simulink model "CMOS_Kernel_Memory_Sync"  (R2023b)
settings: Solver=VariableStepAuto  StartTime=0.0  StopTime=30000000  RelTol=1e-3
values from neighbouring files (symbols this model uses):
  AmountOfPixelsPerScanline = 400    [Kernel_Setup_Script.m]
  AmountOfRamBlocksScanlines = 5    [Kernel_Setup_Script.m]
  AmountOfRamBlocksScanlinesOffset = AmountOfRamBlocksScanlines - 1    (= 4)    [Kernel_Setup_Script.m]
  AmountOfScanlinePixels = 73700    [Kernel_Setup_Script.m]
  AmountOfScanlinePixelsOffset = AmountOfScanlinePixels - 1    (= 73699)    [Kernel_Setup_Script.m]
  AmountOfScanlines = 1100    [Kernel_Setup_Script.m]
  AmountOfScanlinesOffset = AmountOfScanlines - 1    (= 1099)    [Kernel_Setup_Script.m]
  AOPPK_Off = AmountOfPixelsPerScanline - 1    (= 399)    [Kernel_Setup_Script.m]
  AOPPS_Off = AmountOfPixelsPerScanline - 1    (= 399)    [Kernel_Setup_Script.m]
  FramePackOff_0 = FramePackOff_0 - ScanlineFifoCheck    [Kernel_Setup_Script.m]
  FramePackOff_1 = FramePackOff_1 - ScanlineFifoCheck    [Kernel_Setup_Script.m]
  FramePackOff_2 = FramePackOff_2 - ScanlineFifoCheck    [Kernel_Setup_Script.m]
  FramePackOff_3 = FramePackOff_3 - ScanlineFifoCheck    [Kernel_Setup_Script.m]
  FramePackOff_4 = FramePackOff_4 - ScanlineFifoCheck    [Kernel_Setup_Script.m]
  FramePackOff_5 = FramePackOff_5 - ScanlineFifoCheck    [Kernel_Setup_Script.m]
  KernelPackOff_0 = KernelPackOff_0 - KernelBitsPerRow    [Kernel_Setup_Script.m]
  KernelPackOff_1 = KernelPackOff_1 - KernelBitsPerRow    [Kernel_Setup_Script.m]
  KernelPackOff_2 = KernelPackOff_2 - KernelBitsPerRow    [Kernel_Setup_Script.m]
  KernelPackOff_3 = KernelPackOff_3 - KernelBitsPerRow    [Kernel_Setup_Script.m]
  Slice59DownTo48Top = (MsbOffset - (ScanlinePixelBitSizeController*1))    (= 59)    [Kernel_Setup_Script.m]
  Slice71DownTo60Top = (MsbOffset - (ScanlinePixelBitSizeController*0))    (= 71)    [Kernel_Setup_Script.m]
  TotalSectionsForFrames = AmountOfScanlines/AmountOfRamBlocksScanlines    (= 220)    [Kernel_Setup_Script.m]
  UltraRamRows = AmountOfPixelsPerScanline/ScanlineFifoCheck    [Kernel_Setup_Script.m]
  UltraRamRowsCeil = ceil(AmountOfPixelsPerScanline/ScanlineFifoCheck)    [Kernel_Setup_Script.m]
  UltraRamRowsKernel = AmountOfPixelsPerScanline/KernelBitsPerRow    (= 100)    [Kernel_Setup_Script.m]
  UltraRamRowsKernelCeil = ceil(AmountOfPixelsPerScanline/KernelBitsPerRow)    [Kernel_Setup_Script.m]
  UltraRamRowsMemorySectionOffset = UltraRamRowsCeil*AmountOfRamBlocksScanlines    [Kernel_Setup_Script.m]
  UltraRamRowsOffset = UltraRamRowsCeil - 1    [Kernel_Setup_Script.m]
undefined symbols (not defined in the file or in its folder): c, Down, sfvc784, Up, xck26
libraries: hdlBasic x4512, vmcUtilities x1
(part 6 of 39)

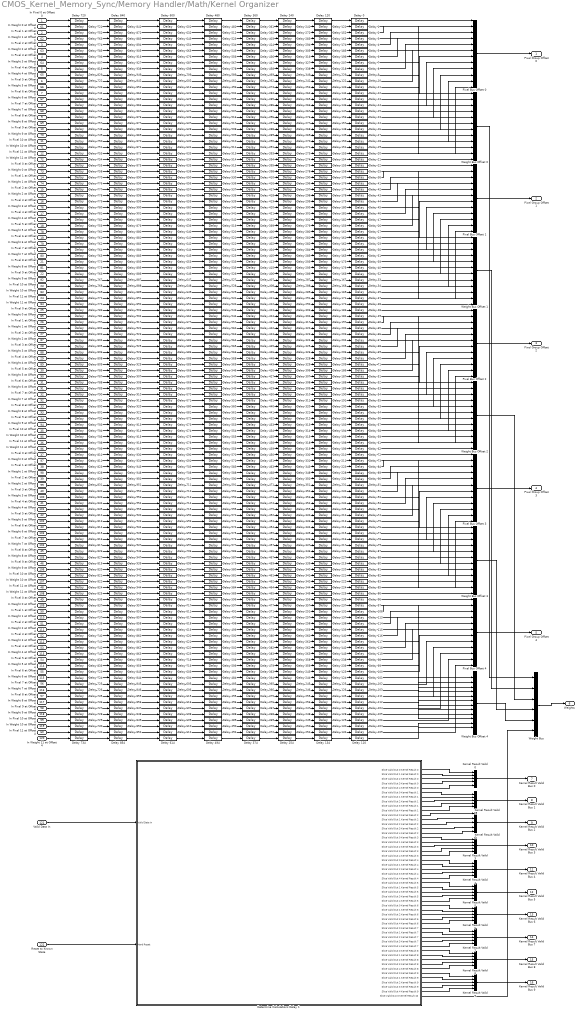
== system CMOS_Kernel_Memory_Sync/Memory Handler/Math/Kernel Organizer ==
  In Pixel 0 at Offset 0 : Inport
  In Pixel 1 at Offset 0 : Inport  Port=2
  In Pixel 2 at Offset 0 : Inport  Port=3
  In Pixel 3 at Offset 0 : Inport  Port=4
  In Pixel 4 at Offset 0 : Inport  Port=5
  In Pixel 5 at Offset 0 : Inport  Port=6
  In Pixel 6 at Offset 0 : Inport  Port=7
  In Pixel 7 at Offset 0 : Inport  Port=8
  In Pixel 8 at Offset 0 : Inport  Port=9
  In Pixel 9 at Offset 0 : Inport  Port=10
  In Pixel 10 at Offset 0 : Inport  Port=11
  In Pixel 11 at Offset 0 : Inport  Port=12
  In Pixel 0 at Offset 1 : Inport  Port=13
  In Pixel 1 at Offset 1 : Inport  Port=14
  In Pixel 2 at Offset 1 : Inport  Port=15
  In Pixel 3 at Offset 1 : Inport  Port=16
  In Pixel 4 at Offset 1 : Inport  Port=17
  In Pixel 5 at Offset 1 : Inport  Port=18
  In Pixel 6 at Offset 1 : Inport  Port=19
  In Pixel 7 at Offset 1 : Inport  Port=20
  In Pixel 8 at Offset 1 : Inport  Port=21
  In Pixel 9 at Offset 1 : Inport  Port=22
  In Pixel 10 at Offset 1 : Inport  Port=23
  In Pixel 11 at Offset 1 : Inport  Port=24
  In Pixel 0 at Offset 2 : Inport  Port=25
  In Pixel 1 at Offset 2 : Inport  Port=26
  In Pixel 2 at Offset 2 : Inport  Port=27
  In Pixel 3 at Offset 2 : Inport  Port=28
  In Pixel 4 at Offset 2 : Inport  Port=29
  In Pixel 5 at Offset 2 : Inport  Port=30
  In Pixel 6 at Offset 2 : Inport  Port=31
  In Pixel 7 at Offset 2 : Inport  Port=32
  In Pixel 8 at Offset 2 : Inport  Port=33
  In Pixel 9 at Offset 2 : Inport  Port=34
  In Pixel 10 at Offset 2 : Inport  Port=35
  In Pixel 11 at Offset 2 : Inport  Port=36
  In Pixel 0 at Offset 3 : Inport  Port=37
  In Pixel 1 at Offset 3 : Inport  Port=38
  In Pixel 2 at Offset 3 : Inport  Port=39
  In Pixel 3 at Offset 3 : Inport  Port=40
  In Pixel 4 at Offset 3 : Inport  Port=41
  In Pixel 5 at Offset 3 : Inport  Port=42
  In Pixel 6 at Offset 3 : Inport  Port=43
  In Pixel 7 at Offset 3 : Inport  Port=44
  In Pixel 8 at Offset 3 : Inport  Port=45
  In Pixel 9 at Offset 3 : Inport  Port=46
  In Pixel 10 at Offset 3 : Inport  Port=47
  In Pixel 11 at Offset 3 : Inport  Port=48
  In Pixel 0 at Offset 4 : Inport  Port=49
  In Pixel 1 at Offset 4 : Inport  Port=50
  In Pixel 2 at Offset 4 : Inport  Port=51
  In Pixel 3 at Offset 4 : Inport  Port=52
  In Pixel 4 at Offset 4 : Inport  Port=53
  In Pixel 5 at Offset 4 : Inport  Port=54
  In Pixel 6 at Offset 4 : Inport  Port=55
  In Pixel 7 at Offset 4 : Inport  Port=56
  In Pixel 8 at Offset 4 : Inport  Port=57
  In Pixel 9 at Offset 4 : Inport  Port=58
  In Pixel 10 at Offset 4 : Inport  Port=59
  In Pixel 11 at Offset 4 : Inport  Port=60
  In Weight 0 at Offset 0 : Inport  Port=61
  In Weight 1 at Offset 0 : Inport  Port=62
  In Weight 2 at Offset 0 : Inport  Port=63
  In Weight 3 at Offset 0 : Inport  Port=64
  In Weight 4 at Offset 0 : Inport  Port=65
  In Weight 5 at Offset 0 : Inport  Port=66
  In Weight 6 at Offset 0 : Inport  Port=67
  In Weight 7 at Offset 0 : Inport  Port=68
  In Weight 8 at Offset 0 : Inport  Port=69
  In Weight 9 at Offset 0 : Inport  Port=70
  In Weight 10 at Offset 0 : Inport  Port=71
  In Weight 11 at Offset 0 : Inport  Port=72
  In Weight 0 at Offset 1 : Inport  Port=73
  In Weight 1 at Offset 1 : Inport  Port=74
  In Weight 2 at Offset 1 : Inport  Port=75
  In Weight 3 at Offset 1 : Inport  Port=76
  In Weight 4 at Offset 1 : Inport  Port=77
  In Weight 5 at Offset 1 : Inport  Port=78
  In Weight 6 at Offset 1 : Inport  Port=79
  In Weight 7 at Offset 1 : Inport  Port=80
  In Weight 8 at Offset 1 : Inport  Port=81
  In Weight 9 at Offset 1 : Inport  Port=82
  In Weight 10 at Offset 1 : Inport  Port=83
  In Weight 11 at Offset 1 : Inport  Port=84
  In Weight 0 at Offset 2 : Inport  Port=85
  In Weight 1 at Offset 2 : Inport  Port=86
  In Weight 2 at Offset 2 : Inport  Port=87
  In Weight 3 at Offset 2 : Inport  Port=88
  In Weight 4 at Offset 2 : Inport  Port=89
  In Weight 5 at Offset 2 : Inport  Port=90
  In Weight 6 at Offset 2 : Inport  Port=91
  In Weight 7 at Offset 2 : Inport  Port=92
  In Weight 8 at Offset 2 : Inport  Port=93
  In Weight 9 at Offset 2 : Inport  Port=94
  In Weight 10 at Offset 2 : Inport  Port=95
  In Weight 11 at Offset 2 : Inport  Port=96
  In Weight 0 at Offset 3 : Inport  Port=97
  In Weight 1 at Offset 3 : Inport  Port=98
  In Weight 2 at Offset 3 : Inport  Port=99
  In Weight 3 at Offset 3 : Inport  Port=100
  In Weight 4 at Offset 3 : Inport  Port=101
  In Weight 5 at Offset 3 : Inport  Port=102
  In Weight 6 at Offset 3 : Inport  Port=103
  In Weight 7 at Offset 3 : Inport  Port=104
  In Weight 8 at Offset 3 : Inport  Port=105
  In Weight 9 at Offset 3 : Inport  Port=106
  In Weight 10 at Offset 3 : Inport  Port=107
  In Weight 11 at Offset 3 : Inport  Port=108
  In Weight 0 at Offset 4 : Inport  Port=109
  In Weight 1 at Offset 4 : Inport  Port=110
  In Weight 2 at Offset 4 : Inport  Port=111
  In Weight 3 at Offset 4 : Inport  Port=112
  In Weight 4 at Offset 4 : Inport  Port=113
  In Weight 5 at Offset 4 : Inport  Port=114
  In Weight 6 at Offset 4 : Inport  Port=115
  In Weight 7 at Offset 4 : Inport  Port=116
  In Weight 8 at Offset 4 : Inport  Port=117
  In Weight 9 at Offset 4 : Inport  Port=118
  In Weight 10 at Offset 4 : Inport  Port=119
  In Weight 11 at Offset 4 : Inport  Port=120
  Valid Data In : Inport  Port=121
  Reset to Known State : Inport  Port=122
  Delay {0..959} (960 alike) : hdlBasic/Delay  rst=off  en=off  latency=1  reg_retiming=off  XmcBlockStatus=1  maskContainerNames=group1  block_type=delay  block_config=sysgen:Delay_config
  Determine Calculations Delay 1 : Subsystem
  Kernel Result Valid {0..9} (10 alike) : BusCreator  Inputs=5
  Pixel Bus Offset {0..4} (5 alike) : BusCreator  Inputs=12
  Weight Bus : BusCreator  Inputs=6
  Weight Bus Offset {0..4} (5 alike) : BusCreator  Inputs=12
  Pixel Group Offset 0 : Outport
  Pixel Group Offset 1 : Outport  Port=2
  Pixel Group Offset 2 : Outport  Port=3
  Pixel Group Offset 3 : Outport  Port=4
  Pixel Group Offset 4 : Outport  Port=5
  Weights : Outport  Port=6
  Kernel Result Valid Bus 0 : Outport  Port=7
  Kernel Result Valid Bus 1 : Outport  Port=8
  Kernel Result Valid Bus 2 : Outport  Port=9
  Kernel Result Valid Bus 3 : Outport  Port=10
  Kernel Result Valid Bus 4 : Outport  Port=11
  Kernel Result Valid Bus 5 : Outport  Port=12
  Kernel Result Valid Bus 6 : Outport  Port=13
  Kernel Result Valid Bus 7 : Outport  Port=14
  Kernel Result Valid Bus 8 : Outport  Port=15
  Kernel Result Valid Bus 9 : Outport  Port=16
  wires:
  Delay 3/1 -> Weight Bus Offset 0/2
  Delay 2/1 -> Pixel Bus Offset 0/2
  Delay 5/1 -> Weight Bus Offset 0/3
  Delay 7/1 -> Weight Bus Offset 0/4
  Delay 6/1 -> Pixel Bus Offset 0/4
  Delay 4/1 -> Pixel Bus Offset 0/3
  Delay 9/1 -> Weight Bus Offset 0/5
  Delay 11/1 -> Weight Bus Offset 0/6
  Delay 10/1 -> Pixel Bus Offset 0/6
  Delay 8/1 -> Pixel Bus Offset 0/5
  Delay 12/1 -> Pixel Bus Offset 0/7
  Delay 13/1 -> Weight Bus Offset 0/7
  Delay 15/1 -> Weight Bus Offset 0/8
  Delay 14/1 -> Pixel Bus Offset 0/8
  Delay 23/1 -> Pixel Bus Offset 0/9
  Delay 16/1 -> Pixel Bus Offset 0/10
  Delay 17/1 -> Weight Bus Offset 0/10
  Delay 19/1 -> Weight Bus Offset 0/11
  Delay 20/1 -> Pixel Bus Offset 0/12
  Delay 21/1 -> Weight Bus Offset 0/12
  Delay 24/1 -> Weight Bus Offset 0/9
  Delay 18/1 -> Pixel Bus Offset 0/11
  Valid Data In/1 -> Determine Calculations Delay 1/1(Valid Data In)
  Determine Calculations Delay 1/1(Slice Valid Out 0 Kernel Result 0) -> Kernel Result Valid 0/1
  Determine Calculations Delay 1/2(Slice Valid Out 1 Kernel Result 0) -> Kernel Result Valid 0/2
  Determine Calculations Delay 1/3(Slice Valid Out 2 Kernel Result 0) -> Kernel Result Valid 0/3
  Determine Calculations Delay 1/4(Slice Valid Out 3 Kernel Result 0) -> Kernel Result Valid 0/4
  Determine Calculations Delay 1/5(Slice Valid Out 4 Kernel Result 0) -> Kernel Result Valid 0/5
  Determine Calculations Delay 1/10(Slice Valid Out 4 Kernel Result 1) -> Kernel Result Valid 1/5
  Determine Calculations Delay 1/6(Slice Valid Out 0 Kernel Result 1) -> Kernel Result Valid 1/1
  Determine Calculations Delay 1/7(Slice Valid Out 1 Kernel Result 1) -> Kernel Result Valid 1/2
  Determine Calculations Delay 1/9(Slice Valid Out 3 Kernel Result 1) -> Kernel Result Valid 1/4
  Determine Calculations Delay 1/8(Slice Valid Out 2 Kernel Result 1) -> Kernel Result Valid 1/3
  Determine Calculations Delay 1/15(Slice Valid Out 4 Kernel Result 2) -> Kernel Result Valid 2/5
  Determine Calculations Delay 1/19(Slice Valid Out 3 Kernel Result 3) -> Kernel Result Valid 3/4
  Determine Calculations Delay 1/17(Slice Valid Out 1 Kernel Result 3) -> Kernel Result Valid 3/2
  Determine Calculations Delay 1/16(Slice Valid Out 0 Kernel Result 3) -> Kernel Result Valid 3/1
  Determine Calculations Delay 1/11(Slice Valid Out 0 Kernel Result 2) -> Kernel Result Valid 2/1
  Determine Calculations Delay 1/12(Slice Valid Out 1 Kernel Result 2) -> Kernel Result Valid 2/2
  Determine Calculations Delay 1/18(Slice Valid Out 2 Kernel Result 3) -> Kernel Result Valid 3/3
  Determine Calculations Delay 1/14(Slice Valid Out 3 Kernel Result 2) -> Kernel Result Valid 2/4
  Determine Calculations Delay 1/20(Slice Valid Out 4 Kernel Result 3) -> Kernel Result Valid 3/5
  Determine Calculations Delay 1/13(Slice Valid Out 2 Kernel Result 2) -> Kernel Result Valid 2/3
  Determine Calculations Delay 1/25(Slice Valid Out 4 Kernel Result 4) -> Kernel Result Valid 4/5
  Determine Calculations Delay 1/21(Slice Valid Out 0 Kernel Result 4) -> Kernel Result Valid 4/1
  Determine Calculations Delay 1/22(Slice Valid Out 1 Kernel Result 4) -> Kernel Result Valid 4/2
  Determine Calculations Delay 1/24(Slice Valid Out 3 Kernel Result 4) -> Kernel Result Valid 4/4
  Determine Calculations Delay 1/23(Slice Valid Out 2 Kernel Result 4) -> Kernel Result Valid 4/3
  Delay 0/1 -> Pixel Bus Offset 0/1
  Delay 1/1 -> Weight Bus Offset 0/1
  Delay 43/1 -> Weight Bus Offset 1/3
  Delay 37/1 -> Pixel Bus Offset 1/12
  Delay 35/1 -> Weight Bus Offset 1/11
  Delay 46/1 -> Pixel Bus Offset 1/5
  Delay 33/1 -> Weight Bus Offset 1/10
  Delay 40/1 -> Weight Bus Offset 1/9
  Delay 28/1 -> Pixel Bus Offset 1/7
  Delay 47/1 -> Weight Bus Offset 1/5
  Delay 22/1 -> Pixel Bus Offset 1/1
  Delay 25/1 -> Weight Bus Offset 1/1
  Delay 38/1 -> Weight Bus Offset 1/12
  Delay 30/1 -> Pixel Bus Offset 1/8
  Delay 36/1 -> Pixel Bus Offset 1/2
  Delay 45/1 -> Weight Bus Offset 1/4
  Delay 42/1 -> Pixel Bus Offset 1/3
  Delay 27/1 -> Weight Bus Offset 1/6
  Delay 39/1 -> Pixel Bus Offset 1/9
  Delay 29/1 -> Weight Bus Offset 1/7
  Delay 34/1 -> Pixel Bus Offset 1/11
  Delay 26/1 -> Pixel Bus Offset 1/6
  Delay 31/1 -> Weight Bus Offset 1/8
  Delay 44/1 -> Pixel Bus Offset 1/4
  Delay 41/1 -> Weight Bus Offset 1/2
  Delay 32/1 -> Pixel Bus Offset 1/10
  Delay 67/1 -> Weight Bus Offset 2/3
  Delay 61/1 -> Pixel Bus Offset 2/12
  Delay 59/1 -> Weight Bus Offset 2/11
  Delay 70/1 -> Pixel Bus Offset 2/5
  Delay 57/1 -> Weight Bus Offset 2/10
  Delay 64/1 -> Weight Bus Offset 2/9
  Delay 52/1 -> Pixel Bus Offset 2/7
  Delay 71/1 -> Weight Bus Offset 2/5
  Delay 48/1 -> Pixel Bus Offset 2/1
  Delay 49/1 -> Weight Bus Offset 2/1
  Delay 62/1 -> Weight Bus Offset 2/12
  Delay 54/1 -> Pixel Bus Offset 2/8
  Delay 60/1 -> Pixel Bus Offset 2/2
  Delay 69/1 -> Weight Bus Offset 2/4
  Delay 66/1 -> Pixel Bus Offset 2/3
  Delay 51/1 -> Weight Bus Offset 2/6
  Delay 63/1 -> Pixel Bus Offset 2/9
  Delay 53/1 -> Weight Bus Offset 2/7
  Delay 58/1 -> Pixel Bus Offset 2/11
  Delay 50/1 -> Pixel Bus Offset 2/6
  Delay 55/1 -> Weight Bus Offset 2/8
  Delay 68/1 -> Pixel Bus Offset 2/4
  Delay 65/1 -> Weight Bus Offset 2/2
  Delay 56/1 -> Pixel Bus Offset 2/10
  Delay 91/1 -> Weight Bus Offset 3/3
  Delay 85/1 -> Pixel Bus Offset 3/12
  Delay 83/1 -> Weight Bus Offset 3/11
  Delay 94/1 -> Pixel Bus Offset 3/5
  Delay 81/1 -> Weight Bus Offset 3/10
  Delay 88/1 -> Weight Bus Offset 3/9
  Delay 76/1 -> Pixel Bus Offset 3/7
  Delay 95/1 -> Weight Bus Offset 3/5
  Delay 72/1 -> Pixel Bus Offset 3/1
  Delay 73/1 -> Weight Bus Offset 3/1
  Delay 86/1 -> Weight Bus Offset 3/12
  Delay 78/1 -> Pixel Bus Offset 3/8
  Delay 84/1 -> Pixel Bus Offset 3/2
  Delay 93/1 -> Weight Bus Offset 3/4
  Delay 90/1 -> Pixel Bus Offset 3/3
  Delay 75/1 -> Weight Bus Offset 3/6
  Delay 87/1 -> Pixel Bus Offset 3/9
  Delay 77/1 -> Weight Bus Offset 3/7
  Delay 82/1 -> Pixel Bus Offset 3/11
  Delay 74/1 -> Pixel Bus Offset 3/6
  Delay 79/1 -> Weight Bus Offset 3/8
  Delay 92/1 -> Pixel Bus Offset 3/4
  Delay 89/1 -> Weight Bus Offset 3/2
  Delay 80/1 -> Pixel Bus Offset 3/10
  Delay 115/1 -> Weight Bus Offset 4/3
  Delay 109/1 -> Pixel Bus Offset 4/12
  Delay 107/1 -> Weight Bus Offset 4/11
  Delay 118/1 -> Pixel Bus Offset 4/5
  Delay 105/1 -> Weight Bus Offset 4/10
  Delay 112/1 -> Weight Bus Offset 4/9
  Delay 100/1 -> Pixel Bus Offset 4/7
  Delay 119/1 -> Weight Bus Offset 4/5
  Delay 96/1 -> Pixel Bus Offset 4/1
  Delay 97/1 -> Weight Bus Offset 4/1
  Delay 110/1 -> Weight Bus Offset 4/12
  Delay 102/1 -> Pixel Bus Offset 4/8
  Delay 108/1 -> Pixel Bus Offset 4/2
  Delay 117/1 -> Weight Bus Offset 4/4
  Delay 114/1 -> Pixel Bus Offset 4/3
  Delay 99/1 -> Weight Bus Offset 4/6
  Delay 111/1 -> Pixel Bus Offset 4/9
  Delay 101/1 -> Weight Bus Offset 4/7
  Delay 106/1 -> Pixel Bus Offset 4/11
  Delay 98/1 -> Pixel Bus Offset 4/6
  Delay 103/1 -> Weight Bus Offset 4/8
  Delay 116/1 -> Pixel Bus Offset 4/4
  Delay 113/1 -> Weight Bus Offset 4/2
  Delay 104/1 -> Pixel Bus Offset 4/10
  Pixel Bus Offset 0/1 -> Pixel Group Offset 0/1
  Pixel Bus Offset 1/1 -> Pixel Group Offset 1/1
  Pixel Bus Offset 2/1 -> Pixel Group Offset 2/1
  Pixel Bus Offset 3/1 -> Pixel Group Offset 3/1
  Pixel Bus Offset 4/1 -> Pixel Group Offset 4/1
  Kernel Result Valid 0/1 -> Kernel Result Valid Bus 0/1
  Kernel Result Valid 1/1 -> Kernel Result Valid Bus 1/1
  Kernel Result Valid 3/1 -> Kernel Result Valid Bus 3/1
  Kernel Result Valid 2/1 -> Kernel Result Valid Bus 2/1
  Kernel Result Valid 4/1 -> Kernel Result Valid Bus 4/1
  Delay 171/1 -> Delay 37/1
  Delay 189/1 -> Delay 53/1
  Delay 190/1 -> Delay 54/1
  Delay 187/1 -> Delay 51/1
  Delay 188/1 -> Delay 52/1
  Delay 137/1 -> Delay 113/1
  Delay 157/1 -> Delay 24/1
  Delay 152/1 -> Delay 2/1
  Delay 150/1 -> Delay 18/1
  Delay 143/1 -> Delay 119/1
  Delay 144/1 -> Delay 12/1
  Delay 145/1 -> Delay 13/1
  Delay 146/1 -> Delay 14/1
  Delay 147/1 -> Delay 15/1
  Delay 148/1 -> Delay 16/1
  Delay 120/1 -> Delay 0/1
  Delay 121/1 -> Delay 1/1
  Delay 122/1 -> Delay 10/1
  Delay 123/1 -> Delay 100/1
  Delay 124/1 -> Delay 101/1
  Delay 126/1 -> Delay 103/1
  Delay 125/1 -> Delay 102/1
  Delay 128/1 -> Delay 105/1
  Delay 129/1 -> Delay 106/1
  Delay 131/1 -> Delay 108/1
  Delay 130/1 -> Delay 107/1
  Delay 134/1 -> Delay 110/1
  Delay 132/1 -> Delay 109/1
  Delay 133/1 -> Delay 11/1
  Delay 151/1 -> Delay 19/1
  Delay 135/1 -> Delay 111/1
  Delay 141/1 -> Delay 117/1
  Delay 136/1 -> Delay 112/1
  Delay 160/1 -> Delay 27/1
  Delay 219/1 -> Delay 80/1
  Delay 185/1 -> Delay 5/1
  Delay 191/1 -> Delay 55/1
  Delay 182/1 -> Delay 47/1
  Delay 183/1 -> Delay 48/1
  Delay 184/1 -> Delay 49/1
  Delay 179/1 -> Delay 44/1
  Delay 178/1 -> Delay 43/1
  Delay 180/1 -> Delay 45/1
  Delay 173/1 -> Delay 39/1
  Delay 174/1 -> Delay 4/1
  Delay 175/1 -> Delay 40/1
  Delay 176/1 -> Delay 41/1
  Delay 177/1 -> Delay 42/1
  Delay 208/1 -> Delay 70/1
  Delay 207/1 -> Delay 7/1
  Delay 200/1 -> Delay 63/1
  Delay 214/1 -> Delay 76/1
  Delay 215/1 -> Delay 77/1
  Delay 217/1 -> Delay 79/1
  Delay 211/1 -> Delay 73/1
  Delay 209/1 -> Delay 71/1
  Delay 210/1 -> Delay 72/1
  Delay 212/1 -> Delay 74/1
  Delay 213/1 -> Delay 75/1
  Delay 192/1 -> Delay 56/1
  Delay 158/1 -> Delay 25/1
  Delay 142/1 -> Delay 118/1
  Delay 138/1 -> Delay 114/1
  Delay 140/1 -> Delay 116/1
  Delay 201/1 -> Delay 64/1
  Delay 203/1 -> Delay 66/1
  Delay 204/1 -> Delay 67/1
  Delay 205/1 -> Delay 68/1
  Delay 206/1 -> Delay 69/1
  Delay 216/1 -> Delay 78/1
  Delay 220/1 -> Delay 81/1
  Delay 199/1 -> Delay 62/1
  Delay 202/1 -> Delay 65/1
  Delay 186/1 -> Delay 50/1
  Delay 193/1 -> Delay 57/1
  Delay 194/1 -> Delay 58/1
  Delay 195/1 -> Delay 59/1
  Delay 196/1 -> Delay 6/1
  Delay 197/1 -> Delay 60/1
  Delay 198/1 -> Delay 61/1
  Delay 226/1 -> Delay 87/1
  Delay 224/1 -> Delay 85/1
  Delay 227/1 -> Delay 88/1
  Delay 225/1 -> Delay 86/1
  Delay 229/1 -> Delay 9/1
  Delay 231/1 -> Delay 91/1
  Delay 228/1 -> Delay 89/1
  Delay 230/1 -> Delay 90/1
  Delay 233/1 -> Delay 93/1
  Delay 232/1 -> Delay 92/1
  Delay 234/1 -> Delay 94/1
  Delay 235/1 -> Delay 95/1
  Delay 238/1 -> Delay 98/1
  Delay 236/1 -> Delay 96/1
  Delay 237/1 -> Delay 97/1
  Delay 239/1 -> Delay 99/1
  Delay 223/1 -> Delay 84/1
  Delay 218/1 -> Delay 8/1
  Delay 172/1 -> Delay 38/1
  Delay 169/1 -> Delay 35/1
  Delay 168/1 -> Delay 34/1
  Delay 221/1 -> Delay 82/1
  Delay 222/1 -> Delay 83/1
  Delay 170/1 -> Delay 36/1
  Delay 161/1 -> Delay 28/1
  Delay 162/1 -> Delay 29/1
  Delay 163/1 -> Delay 3/1
  Delay 165/1 -> Delay 31/1
  Delay 166/1 -> Delay 32/1
  Delay 153/1 -> Delay 20/1
  Delay 154/1 -> Delay 21/1
  Delay 155/1 -> Delay 22/1
  Delay 156/1 -> Delay 23/1
  Delay 159/1 -> Delay 26/1
  Delay 167/1 -> Delay 33/1
  Delay 127/1 -> Delay 104/1
  Delay 149/1 -> Delay 17/1
  Delay 139/1 -> Delay 115/1
  Delay 164/1 -> Delay 30/1
  Delay 181/1 -> Delay 46/1
  Delay 279/1 -> Delay 159/1
  Delay 358/1 -> Delay 238/1
  Delay 357/1 -> Delay 237/1
  Delay 350/1 -> Delay 230/1
  Delay 351/1 -> Delay 231/1
  Delay 353/1 -> Delay 233/1
  Delay 352/1 -> Delay 232/1
  Delay 356/1 -> Delay 236/1
  Delay 320/1 -> Delay 200/1
  Delay 321/1 -> Delay 201/1
  Delay 322/1 -> Delay 202/1
  Delay 323/1 -> Delay 203/1
  Delay 324/1 -> Delay 204/1
  Delay 325/1 -> Delay 205/1
  Delay 326/1 -> Delay 206/1
  Delay 327/1 -> Delay 207/1
  Delay 328/1 -> Delay 208/1
  Delay 329/1 -> Delay 209/1
  Delay 330/1 -> Delay 210/1
  Delay 331/1 -> Delay 211/1
  Delay 333/1 -> Delay 213/1
  Delay 332/1 -> Delay 212/1
  Delay 334/1 -> Delay 214/1
  Delay 336/1 -> Delay 216/1
  Delay 335/1 -> Delay 215/1
  Delay 337/1 -> Delay 217/1
  Delay 338/1 -> Delay 218/1
  Delay 339/1 -> Delay 219/1
  Delay 340/1 -> Delay 220/1
  Delay 342/1 -> Delay 222/1
  Delay 341/1 -> Delay 221/1
  Delay 344/1 -> Delay 224/1
  Delay 343/1 -> Delay 223/1
  Delay 346/1 -> Delay 226/1
  Delay 345/1 -> Delay 225/1
  Delay 347/1 -> Delay 227/1
  Delay 348/1 -> Delay 228/1
  Delay 349/1 -> Delay 229/1
  Delay 274/1 -> Delay 154/1
  Delay 275/1 -> Delay 155/1
  Delay 277/1 -> Delay 157/1
  Delay 280/1 -> Delay 160/1
  Delay 310/1 -> Delay 190/1
  Delay 359/1 -> Delay 239/1
  Delay 276/1 -> Delay 156/1
  Delay 308/1 -> Delay 188/1
  Delay 311/1 -> Delay 191/1
  Delay 312/1 -> Delay 192/1
  Delay 313/1 -> Delay 193/1
  Delay 314/1 -> Delay 194/1
  Delay 315/1 -> Delay 195/1
  Delay 318/1 -> Delay 198/1
  Delay 319/1 -> Delay 199/1
  Delay 281/1 -> Delay 161/1
  Delay 316/1 -> Delay 196/1
  Delay 242/1 -> Delay 122/1
  Delay 241/1 -> Delay 121/1
  Delay 243/1 -> Delay 123/1
  Delay 244/1 -> Delay 124/1
  Delay 245/1 -> Delay 125/1
  Delay 246/1 -> Delay 126/1
  Delay 248/1 -> Delay 128/1
  Delay 247/1 -> Delay 127/1
  Delay 249/1 -> Delay 129/1
  Delay 250/1 -> Delay 130/1
  Delay 251/1 -> Delay 131/1
  Delay 252/1 -> Delay 132/1
  Delay 253/1 -> Delay 133/1
  Delay 255/1 -> Delay 135/1
  Delay 254/1 -> Delay 134/1
  Delay 256/1 -> Delay 136/1
  Delay 258/1 -> Delay 138/1
  Delay 257/1 -> Delay 137/1
  Delay 261/1 -> Delay 141/1
  Delay 259/1 -> Delay 139/1
  Delay 260/1 -> Delay 140/1
  Delay 264/1 -> Delay 144/1
  Delay 263/1 -> Delay 143/1
  Delay 262/1 -> Delay 142/1
  Delay 266/1 -> Delay 146/1
  Delay 267/1 -> Delay 147/1
  Delay 265/1 -> Delay 145/1
  Delay 268/1 -> Delay 148/1
  Delay 270/1 -> Delay 150/1
  Delay 269/1 -> Delay 149/1
  Delay 273/1 -> Delay 153/1
  Delay 271/1 -> Delay 151/1
  Delay 272/1 -> Delay 152/1
  Delay 278/1 -> Delay 158/1
  Delay 240/1 -> Delay 120/1
  Delay 355/1 -> Delay 235/1
  Delay 307/1 -> Delay 187/1
  Delay 297/1 -> Delay 177/1
  Delay 298/1 -> Delay 178/1
  Delay 299/1 -> Delay 179/1
  Delay 300/1 -> Delay 180/1
  Delay 301/1 -> Delay 181/1
  Delay 302/1 -> Delay 182/1
  Delay 303/1 -> Delay 183/1
  Delay 304/1 -> Delay 184/1
  Delay 305/1 -> Delay 185/1
  Delay 306/1 -> Delay 186/1
  Delay 317/1 -> Delay 197/1
  Delay 354/1 -> Delay 234/1
  Delay 309/1 -> Delay 189/1
  Delay 283/1 -> Delay 163/1
  Delay 282/1 -> Delay 162/1
  Delay 285/1 -> Delay 165/1
  Delay 284/1 -> Delay 164/1
  Delay 286/1 -> Delay 166/1
  Delay 287/1 -> Delay 167/1
  Delay 288/1 -> Delay 168/1
  Delay 289/1 -> Delay 169/1
  Delay 291/1 -> Delay 171/1
  Delay 290/1 -> Delay 170/1
  Delay 292/1 -> Delay 172/1
  Delay 293/1 -> Delay 173/1
  Delay 294/1 -> Delay 174/1
  Delay 295/1 -> Delay 175/1
  Delay 296/1 -> Delay 176/1
  Delay 463/1 -> Delay 343/1
  Delay 464/1 -> Delay 344/1
  Delay 465/1 -> Delay 345/1
  Delay 468/1 -> Delay 348/1
  Delay 467/1 -> Delay 347/1
  Delay 466/1 -> Delay 346/1
  Delay 469/1 -> Delay 349/1
  Delay 470/1 -> Delay 350/1
  Delay 477/1 -> Delay 357/1
  Delay 460/1 -> Delay 340/1
  Delay 461/1 -> Delay 341/1
  Delay 462/1 -> Delay 342/1
  Delay 425/1 -> Delay 305/1
  Delay 426/1 -> Delay 306/1
  Delay 424/1 -> Delay 304/1
  Delay 429/1 -> Delay 309/1
  Delay 427/1 -> Delay 307/1
  Delay 428/1 -> Delay 308/1
  Delay 432/1 -> Delay 312/1
  Delay 433/1 -> Delay 313/1
  Delay 431/1 -> Delay 311/1
  Delay 430/1 -> Delay 310/1
  Delay 436/1 -> Delay 316/1
  Delay 435/1 -> Delay 315/1
  Delay 434/1 -> Delay 314/1
  Delay 437/1 -> Delay 317/1
  Delay 438/1 -> Delay 318/1
  Delay 439/1 -> Delay 319/1
  Delay 440/1 -> Delay 320/1
  Delay 441/1 -> Delay 321/1
  Delay 442/1 -> Delay 322/1
  Delay 443/1 -> Delay 323/1
  Delay 423/1 -> Delay 303/1
  Delay 419/1 -> Delay 299/1
  Delay 420/1 -> Delay 300/1
  Delay 418/1 -> Delay 298/1
  Delay 421/1 -> Delay 301/1
  Delay 422/1 -> Delay 302/1
  Delay 389/1 -> Delay 269/1
  Delay 388/1 -> Delay 268/1
  Delay 390/1 -> Delay 270/1
  Delay 391/1 -> Delay 271/1
  Delay 392/1 -> Delay 272/1
  Delay 393/1 -> Delay 273/1
  Delay 394/1 -> Delay 274/1
  Delay 395/1 -> Delay 275/1
  Delay 396/1 -> Delay 276/1
  Delay 398/1 -> Delay 278/1
  Delay 397/1 -> Delay 277/1
  Delay 399/1 -> Delay 279/1
  Delay 400/1 -> Delay 280/1
  Delay 403/1 -> Delay 283/1
  Delay 401/1 -> Delay 281/1
  Delay 402/1 -> Delay 282/1
  Delay 406/1 -> Delay 286/1
  Delay 405/1 -> Delay 285/1
  Delay 404/1 -> Delay 284/1
  Delay 407/1 -> Delay 287/1
  Delay 408/1 -> Delay 288/1
  Delay 409/1 -> Delay 289/1
  Delay 410/1 -> Delay 290/1
  Delay 411/1 -> Delay 291/1
  Delay 412/1 -> Delay 292/1
  Delay 413/1 -> Delay 293/1
  Delay 414/1 -> Delay 294/1
  Delay 416/1 -> Delay 296/1
  Delay 415/1 -> Delay 295/1
  Delay 417/1 -> Delay 297/1
  Delay 360/1 -> Delay 240/1
  Delay 363/1 -> Delay 243/1
  Delay 362/1 -> Delay 242/1
  Delay 361/1 -> Delay 241/1
  Delay 365/1 -> Delay 245/1
  Delay 364/1 -> Delay 244/1
  Delay 367/1 -> Delay 247/1
  Delay 366/1 -> Delay 246/1
  Delay 370/1 -> Delay 250/1
  Delay 369/1 -> Delay 249/1
  Delay 368/1 -> Delay 248/1
  Delay 372/1 -> Delay 252/1
  Delay 371/1 -> Delay 251/1
  Delay 373/1 -> Delay 253/1
  Delay 375/1 -> Delay 255/1
  Delay 374/1 -> Delay 254/1
  Delay 376/1 -> Delay 256/1
  Delay 378/1 -> Delay 258/1
  Delay 377/1 -> Delay 257/1
  Delay 379/1 -> Delay 259/1
  Delay 381/1 -> Delay 261/1
  Delay 380/1 -> Delay 260/1
  Delay 382/1 -> Delay 262/1
  Delay 385/1 -> Delay 265/1
  Delay 384/1 -> Delay 264/1
  Delay 383/1 -> Delay 263/1
  Delay 386/1 -> Delay 266/1
  Delay 387/1 -> Delay 267/1
  Delay 445/1 -> Delay 325/1
  Delay 444/1 -> Delay 324/1
  Delay 448/1 -> Delay 328/1
  Delay 447/1 -> Delay 327/1
  Delay 446/1 -> Delay 326/1
  Delay 449/1 -> Delay 329/1
  Delay 451/1 -> Delay 331/1
  Delay 450/1 -> Delay 330/1
  Delay 452/1 -> Delay 332/1
  Delay 453/1 -> Delay 333/1
  Delay 454/1 -> Delay 334/1
  Delay 455/1 -> Delay 335/1
  Delay 456/1 -> Delay 336/1
  Delay 457/1 -> Delay 337/1
  Delay 459/1 -> Delay 339/1
  Delay 458/1 -> Delay 338/1
  Delay 472/1 -> Delay 352/1
  Delay 471/1 -> Delay 351/1
  Delay 473/1 -> Delay 353/1
  Delay 474/1 -> Delay 354/1
  Delay 478/1 -> Delay 358/1
  Delay 475/1 -> Delay 355/1
  Delay 479/1 -> Delay 359/1
  Delay 476/1 -> Delay 356/1
  In Weight 6 at Offset 0/1 -> Delay 745/1
  In Pixel 7 at Offset 0/1 -> Delay 746/1
  In Weight 7 at Offset 3/1 -> Delay 817/1
  In Weight 11 at Offset 1/1 -> Delay 772/1
  In Weight 4 at Offset 4/1 -> Delay 743/1
  In Pixel 6 at Offset 0/1 -> Delay 744/1
  In Pixel 1 at Offset 1/1 -> Delay 770/1
  In Pixel 3 at Offset 4/1 -> Delay 740/1
  In Pixel 9 at Offset 0/1 -> Delay 748/1
  In Weight 4 at Offset 2/1 -> Delay 809/1
  In Pixel 0 at Offset 3/1 -> Delay 810/1
  In Weight 0 at Offset 3/1 -> Delay 811/1
  In Weight 6 at Offset 3/1 -> Delay 815/1
  In Pixel 5 at Offset 3/1 -> Delay 812/1
  In Pixel 7 at Offset 3/1 -> Delay 816/1
  In Weight 8 at Offset 1/1 -> Delay 775/1
  In Weight 1 at Offset 1/1 -> Delay 776/1
  In Pixel 2 at Offset 1/1 -> Delay 777/1
  In Weight 2 at Offset 1/1 -> Delay 778/1
  In Pixel 4 at Offset 1/1 -> Delay 781/1
  In Weight 3 at Offset 1/1 -> Delay 780/1
  In Pixel 3 at Offset 1/1 -> Delay 779/1
  In Weight 4 at Offset 1/1 -> Delay 782/1
  In Pixel 0 at Offset 2/1 -> Delay 783/1
  In Weight 2 at Offset 0/1 -> Delay 785/1
  In Weight 0 at Offset 2/1 -> Delay 784/1
  In Pixel 6 at Offset 2/1 -> Delay 788/1
  In Weight 6 at Offset 2/1 -> Delay 789/1
  In Weight 5 at Offset 2/1 -> Delay 787/1
  In Pixel 5 at Offset 2/1 -> Delay 786/1
  In Weight 7 at Offset 2/1 -> Delay 791/1
  In Pixel 7 at Offset 2/1 -> Delay 790/1
  In Pixel 9 at Offset 2/1 -> Delay 792/1
  In Weight 9 at Offset 2/1 -> Delay 793/1
  In Pixel 10 at Offset 2/1 -> Delay 794/1
  In Weight 10 at Offset 2/1 -> Delay 795/1
  In Pixel 3 at Offset 0/1 -> Delay 796/1
  In Pixel 11 at Offset 2/1 -> Delay 798/1
  In Pixel 1 at Offset 2/1 -> Delay 797/1
  In Weight 1 at Offset 2/1 -> Delay 802/1
  In Weight 11 at Offset 2/1 -> Delay 799/1
  In Weight 8 at Offset 2/1 -> Delay 801/1
  In Pixel 8 at Offset 2/1 -> Delay 800/1
  In Pixel 2 at Offset 2/1 -> Delay 803/1
  In Weight 2 at Offset 2/1 -> Delay 804/1
  In Weight 3 at Offset 2/1 -> Delay 806/1
  In Weight 3 at Offset 0/1 -> Delay 807/1
  In Pixel 3 at Offset 2/1 -> Delay 805/1
  In Pixel 4 at Offset 2/1 -> Delay 808/1
  In Weight 5 at Offset 3/1 -> Delay 813/1
  In Pixel 4 at Offset 0/1 -> Delay 818/1
  In Pixel 2 at Offset 0/1 -> Delay 774/1
  In Weight 9 at Offset 0/1 -> Delay 749/1
  In Pixel 10 at Offset 0/1 -> Delay 750/1
  In Pixel 1 at Offset 0/1 -> Delay 752/1
  In Weight 10 at Offset 0/1 -> Delay 751/1
  In Pixel 11 at Offset 0/1 -> Delay 753/1
  In Weight 11 at Offset 0/1 -> Delay 754/1
  In Pixel 0 at Offset 1/1 -> Delay 755/1
  In Weight 8 at Offset 0/1 -> Delay 757/1
  In Pixel 8 at Offset 0/1 -> Delay 756/1
  In Weight 0 at Offset 1/1 -> Delay 758/1
  In Pixel 6 at Offset 1/1 -> Delay 761/1
  In Pixel 5 at Offset 1/1 -> Delay 759/1
  In Weight 5 at Offset 1/1 -> Delay 760/1
  In Weight 6 at Offset 1/1 -> Delay 762/1
  In Weight 1 at Offset 0/1 -> Delay 763/1
  In Pixel 7 at Offset 1/1 -> Delay 764/1
  In Weight 7 at Offset 1/1 -> Delay 765/1
  In Pixel 9 at Offset 1/1 -> Delay 766/1
  In Weight 9 at Offset 1/1 -> Delay 767/1
  In Pixel 10 at Offset 1/1 -> Delay 768/1
  In Weight 10 at Offset 1/1 -> Delay 769/1
  In Pixel 11 at Offset 1/1 -> Delay 771/1
  In Weight 6 at Offset 4/1 -> Delay 724/1
  In Pixel 7 at Offset 4/1 -> Delay 725/1
  In Weight 7 at Offset 4/1 -> Delay 726/1
  In Pixel 9 at Offset 4/1 -> Delay 727/1
  In Weight 9 at Offset 4/1 -> Delay 728/1
  In Pixel 10 at Offset 4/1 -> Delay 729/1
  In Weight 10 at Offset 4/1 -> Delay 730/1
  In Pixel 1 at Offset 4/1 -> Delay 731/1
  In Pixel 4 at Offset 4/1 -> Delay 742/1
  In Weight 2 at Offset 4/1 -> Delay 739/1
  In Weight 7 at Offset 0/1 -> Delay 747/1
  In Pixel 0 at Offset 0/1 -> Delay 720/1
  In Weight 0 at Offset 0/1 -> Delay 721/1
  In Pixel 5 at Offset 0/1 -> Delay 722/1
  In Pixel 6 at Offset 4/1 -> Delay 723/1
  In Weight 3 at Offset 3/1 -> Delay 833/1
  In Pixel 4 at Offset 3/1 -> Delay 834/1
  In Weight 4 at Offset 3/1 -> Delay 835/1
  In Pixel 0 at Offset 4/1 -> Delay 836/1
  In Weight 0 at Offset 4/1 -> Delay 837/1
  In Pixel 5 at Offset 4/1 -> Delay 838/1
  In Weight 5 at Offset 4/1 -> Delay 839/1
  In Pixel 10 at Offset 3/1 -> Delay 821/1
  In Weight 10 at Offset 3/1 -> Delay 822/1
  In Weight 9 at Offset 3/1 -> Delay 820/1
  In Pixel 9 at Offset 3/1 -> Delay 819/1
  In Pixel 1 at Offset 3/1 -> Delay 823/1
  In Pixel 11 at Offset 3/1 -> Delay 824/1
  In Weight 11 at Offset 3/1 -> Delay 825/1
  In Pixel 8 at Offset 3/1 -> Delay 826/1
  In Weight 1 at Offset 3/1 -> Delay 828/1
  In Weight 8 at Offset 3/1 -> Delay 827/1
  In Pixel 2 at Offset 3/1 -> Delay 830/1
  In Weight 4 at Offset 0/1 -> Delay 829/1
  In Weight 2 at Offset 3/1 -> Delay 831/1
  In Pixel 3 at Offset 3/1 -> Delay 832/1
  In Weight 3 at Offset 4/1 -> Delay 741/1
  In Pixel 11 at Offset 4/1 -> Delay 732/1
  In Weight 5 at Offset 0/1 -> Delay 733/1
  In Weight 11 at Offset 4/1 -> Delay 734/1
  In Pixel 8 at Offset 4/1 -> Delay 735/1
  In Weight 8 at Offset 4/1 -> Delay 736/1
  In Weight 1 at Offset 4/1 -> Delay 737/1
  In Pixel 2 at Offset 4/1 -> Delay 738/1
  In Pixel 8 at Offset 1/1 -> Delay 773/1
  In Pixel 6 at Offset 3/1 -> Delay 814/1
  Determine Calculations Delay 1/30(Slice Valid Out 4 Kernel Result 5) -> Kernel Result Valid 5/5
  Kernel Result Valid 5/1 -> Kernel Result Valid Bus 5/1
  Determine Calculations Delay 1/27(Slice Valid Out 1 Kernel Result 5) -> Kernel Result Valid 5/2
  Determine Calculations Delay 1/26(Slice Valid Out 0 Kernel Result 5) -> Kernel Result Valid 5/1
  Determine Calculations Delay 1/29(Slice Valid Out 3 Kernel Result 5) -> Kernel Result Valid 5/4
  Determine Calculations Delay 1/28(Slice Valid Out 2 Kernel Result 5) -> Kernel Result Valid 5/3
  Determine Calculations Delay 1/35(Slice Valid Out 4 Kernel Result 6) -> Kernel Result Valid 6/5
  Kernel Result Valid 6/1 -> Kernel Result Valid Bus 6/1
  Determine Calculations Delay 1/32(Slice Valid Out 1 Kernel Result 6) -> Kernel Result Valid 6/2
  Determine Calculations Delay 1/31(Slice Valid Out 0 Kernel Result 6) -> Kernel Result Valid 6/1
  Determine Calculations Delay 1/34(Slice Valid Out 3 Kernel Result 6) -> Kernel Result Valid 6/4
  Determine Calculations Delay 1/33(Slice Valid Out 2 Kernel Result 6) -> Kernel Result Valid 6/3
  Determine Calculations Delay 1/40(Slice Valid Out 4 Kernel Result 7) -> Kernel Result Valid 7/5
  Kernel Result Valid 7/1 -> Kernel Result Valid Bus 7/1
  Determine Calculations Delay 1/37(Slice Valid Out 1 Kernel Result 7) -> Kernel Result Valid 7/2
  Determine Calculations Delay 1/36(Slice Valid Out 0 Kernel Result 7) -> Kernel Result Valid 7/1
  Determine Calculations Delay 1/39(Slice Valid Out 3 Kernel Result 7) -> Kernel Result Valid 7/4
  Determine Calculations Delay 1/38(Slice Valid Out 2 Kernel Result 7) -> Kernel Result Valid 7/3
  Determine Calculations Delay 1/45(Slice Valid Out 4 Kernel Result 8) -> Kernel Result Valid 8/5
  Kernel Result Valid 8/1 -> Kernel Result Valid Bus 8/1
  Determine Calculations Delay 1/42(Slice Valid Out 1 Kernel Result 8) -> Kernel Result Valid 8/2
  Determine Calculations Delay 1/41(Slice Valid Out 0 Kernel Result 8) -> Kernel Result Valid 8/1
  Determine Calculations Delay 1/44(Slice Valid Out 3 Kernel Result 8) -> Kernel Result Valid 8/4
  Determine Calculations Delay 1/43(Slice Valid Out 2 Kernel Result 8) -> Kernel Result Valid 8/3
  Determine Calculations Delay 1/50(Slice Valid Out 4 Kernel Result 9) -> Kernel Result Valid 9/5
  Kernel Result Valid 9/1 -> Kernel Result Valid Bus 9/1
  Determine Calculations Delay 1/47(Slice Valid Out 1 Kernel Result 9) -> Kernel Result Valid 9/2
  Determine Calculations Delay 1/46(Slice Valid Out 0 Kernel Result 9) -> Kernel Result Valid 9/1
  Determine Calculations Delay 1/49(Slice Valid Out 3 Kernel Result 9) -> Kernel Result Valid 9/4
  Determine Calculations Delay 1/48(Slice Valid Out 2 Kernel Result 9) -> Kernel Result Valid 9/3
  Weight Bus/1 -> Weights/1
  Weight Bus Offset 4/1 -> Weight Bus/5
  Weight Bus Offset 3/1 -> Weight Bus/4
  Weight Bus Offset 2/1 -> Weight Bus/3
  Weight Bus Offset 1/1 -> Weight Bus/2
  Weight Bus Offset 0/1 -> Weight Bus/1
  Delay 489/1 -> Delay 369/1
  Delay 491/1 -> Delay 371/1
  Delay 490/1 -> Delay 370/1
  Delay 492/1 -> Delay 372/1
  Delay 480/1 -> Delay 360/1
  Delay 481/1 -> Delay 361/1
  Delay 482/1 -> Delay 362/1
  Delay 483/1 -> Delay 363/1
  Delay 484/1 -> Delay 364/1
  Delay 485/1 -> Delay 365/1
  Delay 486/1 -> Delay 366/1
  Delay 488/1 -> Delay 368/1
  Delay 487/1 -> Delay 367/1
  Delay 526/1 -> Delay 406/1
  Delay 524/1 -> Delay 404/1
  Delay 523/1 -> Delay 403/1
  Delay 525/1 -> Delay 405/1
  Delay 529/1 -> Delay 409/1
  Delay 527/1 -> Delay 407/1
  Delay 528/1 -> Delay 408/1
  Delay 496/1 -> Delay 376/1
  Delay 493/1 -> Delay 373/1
  Delay 495/1 -> Delay 375/1
  Delay 494/1 -> Delay 374/1
  Delay 500/1 -> Delay 380/1
  Delay 498/1 -> Delay 378/1
  Delay 499/1 -> Delay 379/1
  Delay 497/1 -> Delay 377/1
  Delay 504/1 -> Delay 384/1
  Delay 503/1 -> Delay 383/1
  Delay 501/1 -> Delay 381/1
  Delay 502/1 -> Delay 382/1
  Delay 508/1 -> Delay 388/1
  Delay 505/1 -> Delay 385/1
  Delay 507/1 -> Delay 387/1
  Delay 506/1 -> Delay 386/1
  Delay 512/1 -> Delay 392/1
  Delay 509/1 -> Delay 389/1
  Delay 511/1 -> Delay 391/1
  Delay 510/1 -> Delay 390/1
  Delay 513/1 -> Delay 393/1
  Delay 514/1 -> Delay 394/1
  Delay 515/1 -> Delay 395/1
  Delay 516/1 -> Delay 396/1
  Delay 517/1 -> Delay 397/1
  Delay 520/1 -> Delay 400/1
  Delay 519/1 -> Delay 399/1
  Delay 518/1 -> Delay 398/1
  Delay 521/1 -> Delay 401/1
  Delay 522/1 -> Delay 402/1
  Delay 531/1 -> Delay 411/1
  Delay 530/1 -> Delay 410/1
  Delay 533/1 -> Delay 413/1
  Delay 532/1 -> Delay 412/1
  Delay 536/1 -> Delay 416/1
  Delay 537/1 -> Delay 417/1
  Delay 534/1 -> Delay 414/1
  Delay 535/1 -> Delay 415/1
  Delay 541/1 -> Delay 421/1
  Delay 539/1 -> Delay 419/1
  Delay 540/1 -> Delay 420/1
  Delay 538/1 -> Delay 418/1
  Delay 545/1 -> Delay 425/1
  Delay 542/1 -> Delay 422/1
  Delay 544/1 -> Delay 424/1
  Delay 543/1 -> Delay 423/1
  Delay 549/1 -> Delay 429/1
  Delay 546/1 -> Delay 426/1
  Delay 547/1 -> Delay 427/1
  Delay 548/1 -> Delay 428/1
  Delay 550/1 -> Delay 430/1
  Delay 551/1 -> Delay 431/1
  Delay 552/1 -> Delay 432/1
  Delay 553/1 -> Delay 433/1
  Delay 557/1 -> Delay 437/1
  Delay 554/1 -> Delay 434/1
  Delay 555/1 -> Delay 435/1
  Delay 556/1 -> Delay 436/1
  Delay 561/1 -> Delay 441/1
  Delay 560/1 -> Delay 440/1
  Delay 558/1 -> Delay 438/1
  Delay 559/1 -> Delay 439/1
  Delay 564/1 -> Delay 444/1
  Delay 562/1 -> Delay 442/1
  Delay 563/1 -> Delay 443/1
  Delay 566/1 -> Delay 446/1
  Delay 565/1 -> Delay 445/1
  Delay 568/1 -> Delay 448/1
  Delay 567/1 -> Delay 447/1
  Delay 571/1 -> Delay 451/1
  Delay 569/1 -> Delay 449/1
  Delay 572/1 -> Delay 452/1
  Delay 570/1 -> Delay 450/1
  Delay 575/1 -> Delay 455/1
  Delay 573/1 -> Delay 453/1
  Delay 576/1 -> Delay 456/1
  Delay 574/1 -> Delay 454/1
  Delay 578/1 -> Delay 458/1
  Delay 579/1 -> Delay 459/1
  Delay 577/1 -> Delay 457/1
  Delay 581/1 -> Delay 461/1
  Delay 580/1 -> Delay 460/1
  Delay 582/1 -> Delay 462/1
  Delay 585/1 -> Delay 465/1
  Delay 583/1 -> Delay 463/1
  Delay 586/1 -> Delay 466/1
  Delay 584/1 -> Delay 464/1
  Delay 590/1 -> Delay 470/1
  Delay 588/1 -> Delay 468/1
  Delay 589/1 -> Delay 469/1
  Delay 587/1 -> Delay 467/1
  Delay 594/1 -> Delay 474/1
  Delay 592/1 -> Delay 472/1
  Delay 593/1 -> Delay 473/1
  Delay 591/1 -> Delay 471/1
  Delay 597/1 -> Delay 477/1
  Delay 596/1 -> Delay 476/1
  Delay 598/1 -> Delay 478/1
  Delay 595/1 -> Delay 475/1
  Delay 599/1 -> Delay 479/1
  Delay 670/1 -> Delay 550/1
  Delay 652/1 -> Delay 532/1
  Delay 656/1 -> Delay 536/1
  Delay 657/1 -> Delay 537/1
  Delay 658/1 -> Delay 538/1
  Delay 659/1 -> Delay 539/1
  Delay 660/1 -> Delay 540/1
  Delay 671/1 -> Delay 551/1
  Delay 661/1 -> Delay 541/1
  Delay 662/1 -> Delay 542/1
  Delay 663/1 -> Delay 543/1
  Delay 664/1 -> Delay 544/1
  Delay 665/1 -> Delay 545/1
  Delay 666/1 -> Delay 546/1
  Delay 667/1 -> Delay 547/1
  Delay 668/1 -> Delay 548/1
  Delay 669/1 -> Delay 549/1
  Delay 653/1 -> Delay 533/1
  Delay 621/1 -> Delay 501/1
  Delay 622/1 -> Delay 502/1
  Delay 623/1 -> Delay 503/1
  Delay 624/1 -> Delay 504/1
  Delay 625/1 -> Delay 505/1
  Delay 626/1 -> Delay 506/1
  Delay 627/1 -> Delay 507/1
  Delay 628/1 -> Delay 508/1
  Delay 629/1 -> Delay 509/1
  Delay 630/1 -> Delay 510/1
  Delay 632/1 -> Delay 512/1
  Delay 634/1 -> Delay 514/1
  Delay 631/1 -> Delay 511/1
  Delay 633/1 -> Delay 513/1
  Delay 635/1 -> Delay 515/1
  Delay 637/1 -> Delay 517/1
  Delay 636/1 -> Delay 516/1
  Delay 638/1 -> Delay 518/1
  Delay 640/1 -> Delay 520/1
  Delay 641/1 -> Delay 521/1
  Delay 639/1 -> Delay 519/1
  Delay 642/1 -> Delay 522/1
  Delay 643/1 -> Delay 523/1
  Delay 645/1 -> Delay 525/1
  Delay 644/1 -> Delay 524/1
  Delay 648/1 -> Delay 528/1
  Delay 646/1 -> Delay 526/1
  Delay 647/1 -> Delay 527/1
  Delay 651/1 -> Delay 531/1
  Delay 649/1 -> Delay 529/1
  Delay 655/1 -> Delay 535/1
  Delay 650/1 -> Delay 530/1
  Delay 672/1 -> Delay 552/1
  Delay 613/1 -> Delay 493/1
  Delay 612/1 -> Delay 492/1
  Delay 614/1 -> Delay 494/1
  Delay 616/1 -> Delay 496/1
  Delay 617/1 -> Delay 497/1
  Delay 615/1 -> Delay 495/1
  Delay 618/1 -> Delay 498/1
  Delay 619/1 -> Delay 499/1
  Delay 620/1 -> Delay 500/1
  Delay 698/1 -> Delay 578/1
  Delay 697/1 -> Delay 577/1
  Delay 601/1 -> Delay 481/1
  Delay 600/1 -> Delay 480/1
  Delay 602/1 -> Delay 482/1
  Delay 606/1 -> Delay 486/1
  Delay 603/1 -> Delay 483/1
  Delay 605/1 -> Delay 485/1
  Delay 604/1 -> Delay 484/1
  Delay 609/1 -> Delay 489/1
  Delay 608/1 -> Delay 488/1
  Delay 607/1 -> Delay 487/1
  Delay 610/1 -> Delay 490/1
  Delay 611/1 -> Delay 491/1
  Delay 654/1 -> Delay 534/1
  Delay 701/1 -> Delay 581/1
  Delay 700/1 -> Delay 580/1
  Delay 699/1 -> Delay 579/1
  Delay 702/1 -> Delay 582/1
  Delay 704/1 -> Delay 584/1
  Delay 703/1 -> Delay 583/1
  Delay 705/1 -> Delay 585/1
  Delay 708/1 -> Delay 588/1
  Delay 707/1 -> Delay 587/1
  Delay 709/1 -> Delay 589/1
  Delay 706/1 -> Delay 586/1
  Delay 712/1 -> Delay 592/1
  Delay 711/1 -> Delay 591/1
  Delay 710/1 -> Delay 590/1
  Delay 713/1 -> Delay 593/1
  Delay 715/1 -> Delay 595/1
  Delay 716/1 -> Delay 596/1
  Delay 714/1 -> Delay 594/1
  Delay 717/1 -> Delay 597/1
  Delay 719/1 -> Delay 599/1
  Delay 718/1 -> Delay 598/1
  Delay 679/1 -> Delay 559/1
  Delay 680/1 -> Delay 560/1
  Delay 682/1 -> Delay 562/1
  Delay 681/1 -> Delay 561/1
  Delay 683/1 -> Delay 563/1
  Delay 684/1 -> Delay 564/1
  Delay 686/1 -> Delay 566/1
  Delay 687/1 -> Delay 567/1
  Delay 685/1 -> Delay 565/1
  Delay 688/1 -> Delay 568/1
  Delay 689/1 -> Delay 569/1
  Delay 690/1 -> Delay 570/1
  Delay 692/1 -> Delay 572/1
  Delay 691/1 -> Delay 571/1
  Delay 695/1 -> Delay 575/1
  Delay 696/1 -> Delay 576/1
  Delay 694/1 -> Delay 574/1
  Delay 693/1 -> Delay 573/1
  Delay 674/1 -> Delay 554/1
  Delay 673/1 -> Delay 553/1
  Delay 675/1 -> Delay 555/1
  Delay 676/1 -> Delay 556/1
  Delay 677/1 -> Delay 557/1
  Delay 678/1 -> Delay 558/1
  Determine Calculations Delay 1/51(Slice Valid Out 0 Kernel Result 10) -> Weight Bus/6
  Reset to Known State/1 -> Determine Calculations Delay 1/2(Hard Reset)
  Delay 794/1 -> Delay 914/1
  Delay 740/1 -> Delay 860/1
  Delay 742/1 -> Delay 862/1
  Delay 741/1 -> Delay 861/1
  Delay 744/1 -> Delay 864/1
  Delay 743/1 -> Delay 863/1
  Delay 746/1 -> Delay 866/1
  Delay 745/1 -> Delay 865/1
  Delay 748/1 -> Delay 868/1
  Delay 747/1 -> Delay 867/1
  Delay 749/1 -> Delay 869/1
  Delay 750/1 -> Delay 870/1
  Delay 751/1 -> Delay 871/1
  Delay 752/1 -> Delay 872/1
  Delay 789/1 -> Delay 909/1
  Delay 821/1 -> Delay 941/1
  Delay 721/1 -> Delay 841/1
  Delay 722/1 -> Delay 842/1
  Delay 723/1 -> Delay 843/1
  Delay 725/1 -> Delay 845/1
  Delay 724/1 -> Delay 844/1
  Delay 727/1 -> Delay 847/1
  Delay 726/1 -> Delay 846/1
  Delay 728/1 -> Delay 848/1
  Delay 730/1 -> Delay 850/1
  Delay 729/1 -> Delay 849/1
  Delay 731/1 -> Delay 851/1
  Delay 735/1 -> Delay 855/1
  Delay 734/1 -> Delay 854/1
  Delay 732/1 -> Delay 852/1
  Delay 733/1 -> Delay 853/1
  Delay 738/1 -> Delay 858/1
  Delay 737/1 -> Delay 857/1
  Delay 736/1 -> Delay 856/1
  Delay 739/1 -> Delay 859/1
  Delay 798/1 -> Delay 918/1
  Delay 775/1 -> Delay 895/1
  Delay 774/1 -> Delay 894/1
  Delay 776/1 -> Delay 896/1
  Delay 777/1 -> Delay 897/1
  Delay 778/1 -> Delay 898/1
  Delay 779/1 -> Delay 899/1
  Delay 780/1 -> Delay 900/1
  Delay 781/1 -> Delay 901/1
  Delay 782/1 -> Delay 902/1
  Delay 783/1 -> Delay 903/1
  Delay 804/1 -> Delay 924/1
  Delay 788/1 -> Delay 908/1
  Delay 793/1 -> Delay 913/1
  Delay 772/1 -> Delay 892/1
  Delay 773/1 -> Delay 893/1
  Delay 787/1 -> Delay 907/1
  Delay 792/1 -> Delay 912/1
  Delay 764/1 -> Delay 884/1
  Delay 765/1 -> Delay 885/1
  Delay 766/1 -> Delay 886/1
  Delay 767/1 -> Delay 887/1
  Delay 768/1 -> Delay 888/1
  Delay 769/1 -> Delay 889/1
  Delay 770/1 -> Delay 890/1
  Delay 771/1 -> Delay 891/1
  Delay 817/1 -> Delay 937/1
  Delay 790/1 -> Delay 910/1
  Delay 801/1 -> Delay 921/1
  Delay 797/1 -> Delay 917/1
  Delay 786/1 -> Delay 906/1
  Delay 802/1 -> Delay 922/1
  Delay 799/1 -> Delay 919/1
  Delay 820/1 -> Delay 940/1
  Delay 819/1 -> Delay 939/1
  Delay 791/1 -> Delay 911/1
  Delay 720/1 -> Delay 840/1
  Delay 805/1 -> Delay 925/1
  Delay 806/1 -> Delay 926/1
  Delay 809/1 -> Delay 929/1
  Delay 808/1 -> Delay 928/1
  Delay 807/1 -> Delay 927/1
  Delay 811/1 -> Delay 931/1
  Delay 812/1 -> Delay 932/1
  Delay 810/1 -> Delay 930/1
  Delay 813/1 -> Delay 933/1
  Delay 814/1 -> Delay 934/1
  Delay 815/1 -> Delay 935/1
  Delay 816/1 -> Delay 936/1
  Delay 818/1 -> Delay 938/1
  Delay 825/1 -> Delay 945/1
  Delay 826/1 -> Delay 946/1
  Delay 827/1 -> Delay 947/1
  Delay 828/1 -> Delay 948/1
  Delay 829/1 -> Delay 949/1
  Delay 830/1 -> Delay 950/1
  Delay 832/1 -> Delay 952/1
  Delay 831/1 -> Delay 951/1
  Delay 833/1 -> Delay 953/1
  Delay 834/1 -> Delay 954/1
  Delay 835/1 -> Delay 955/1
  Delay 836/1 -> Delay 956/1
  Delay 837/1 -> Delay 957/1
  Delay 838/1 -> Delay 958/1
  Delay 839/1 -> Delay 959/1
  Delay 824/1 -> Delay 944/1
  Delay 822/1 -> Delay 942/1
  Delay 823/1 -> Delay 943/1
  Delay 785/1 -> Delay 905/1
  Delay 784/1 -> Delay 904/1
  Delay 795/1 -> Delay 915/1
  Delay 796/1 -> Delay 916/1
  Delay 753/1 -> Delay 873/1
  Delay 754/1 -> Delay 874/1
  Delay 755/1 -> Delay 875/1
  Delay 756/1 -> Delay 876/1
  Delay 757/1 -> Delay 877/1
  Delay 759/1 -> Delay 879/1
  Delay 758/1 -> Delay 878/1
  Delay 762/1 -> Delay 882/1
  Delay 761/1 -> Delay 881/1
  Delay 760/1 -> Delay 880/1
  Delay 800/1 -> Delay 920/1
  Delay 763/1 -> Delay 883/1
  Delay 803/1 -> Delay 923/1
  Delay 924/1 -> Delay 684/1
  Delay 925/1 -> Delay 685/1
  Delay 926/1 -> Delay 686/1
  Delay 927/1 -> Delay 687/1
  Delay 928/1 -> Delay 688/1
  Delay 929/1 -> Delay 689/1
  Delay 930/1 -> Delay 690/1
  Delay 931/1 -> Delay 691/1
  Delay 932/1 -> Delay 692/1
  Delay 933/1 -> Delay 693/1
  Delay 934/1 -> Delay 694/1
  Delay 935/1 -> Delay 695/1
  Delay 936/1 -> Delay 696/1
  Delay 848/1 -> Delay 608/1
  Delay 847/1 -> Delay 607/1
  Delay 849/1 -> Delay 609/1
  Delay 850/1 -> Delay 610/1
  Delay 851/1 -> Delay 611/1
  Delay 852/1 -> Delay 612/1
  Delay 853/1 -> Delay 613/1
  Delay 854/1 -> Delay 614/1
  Delay 855/1 -> Delay 615/1
  Delay 856/1 -> Delay 616/1
  Delay 857/1 -> Delay 617/1
  Delay 858/1 -> Delay 618/1
  Delay 840/1 -> Delay 600/1
  Delay 841/1 -> Delay 601/1
  Delay 844/1 -> Delay 604/1
  Delay 842/1 -> Delay 602/1
  Delay 843/1 -> Delay 603/1
  Delay 846/1 -> Delay 606/1
  Delay 845/1 -> Delay 605/1
  Delay 908/1 -> Delay 668/1
  Delay 907/1 -> Delay 667/1
  Delay 909/1 -> Delay 669/1
  Delay 910/1 -> Delay 670/1
  Delay 911/1 -> Delay 671/1
  Delay 912/1 -> Delay 672/1
  Delay 913/1 -> Delay 673/1
  Delay 914/1 -> Delay 674/1
  Delay 916/1 -> Delay 676/1
  Delay 915/1 -> Delay 675/1
  Delay 917/1 -> Delay 677/1
  Delay 920/1 -> Delay 680/1
  Delay 919/1 -> Delay 679/1
  Delay 918/1 -> Delay 678/1
  Delay 921/1 -> Delay 681/1
  Delay 922/1 -> Delay 682/1
  Delay 923/1 -> Delay 683/1
  Delay 939/1 -> Delay 699/1
  Delay 940/1 -> Delay 700/1
  Delay 941/1 -> Delay 701/1
  Delay 942/1 -> Delay 702/1
  Delay 943/1 -> Delay 703/1
  Delay 944/1 -> Delay 704/1
  Delay 945/1 -> Delay 705/1
  Delay 946/1 -> Delay 706/1
  Delay 937/1 -> Delay 697/1
  Delay 938/1 -> Delay 698/1
  Delay 897/1 -> Delay 657/1
  Delay 898/1 -> Delay 658/1
  Delay 899/1 -> Delay 659/1
  Delay 900/1 -> Delay 660/1
  Delay 901/1 -> Delay 661/1
  Delay 903/1 -> Delay 663/1
  Delay 902/1 -> Delay 662/1
  Delay 904/1 -> Delay 664/1
  Delay 905/1 -> Delay 665/1
  Delay 906/1 -> Delay 666/1
  Delay 884/1 -> Delay 644/1
  Delay 883/1 -> Delay 643/1
  Delay 885/1 -> Delay 645/1
  Delay 887/1 -> Delay 647/1
  Delay 886/1 -> Delay 646/1
  Delay 888/1 -> Delay 648/1
  Delay 890/1 -> Delay 650/1
  Delay 891/1 -> Delay 651/1
  Delay 889/1 -> Delay 649/1
  Delay 892/1 -> Delay 652/1
  Delay 893/1 -> Delay 653/1
  Delay 894/1 -> Delay 654/1
  Delay 896/1 -> Delay 656/1
  Delay 895/1 -> Delay 655/1
  Delay 955/1 -> Delay 715/1
  Delay 956/1 -> Delay 716/1
  Delay 958/1 -> Delay 718/1
  Delay 957/1 -> Delay 717/1
  Delay 959/1 -> Delay 719/1
  Delay 880/1 -> Delay 640/1
  Delay 881/1 -> Delay 641/1
  Delay 882/1 -> Delay 642/1
  Delay 859/1 -> Delay 619/1
  Delay 860/1 -> Delay 620/1
  Delay 864/1 -> Delay 624/1
  Delay 861/1 -> Delay 621/1
  Delay 862/1 -> Delay 622/1
  Delay 863/1 -> Delay 623/1
  Delay 866/1 -> Delay 626/1
  Delay 867/1 -> Delay 627/1
  Delay 865/1 -> Delay 625/1
  Delay 868/1 -> Delay 628/1
  Delay 869/1 -> Delay 629/1
  Delay 872/1 -> Delay 632/1
  Delay 873/1 -> Delay 633/1
  Delay 871/1 -> Delay 631/1
  Delay 870/1 -> Delay 630/1
  Delay 875/1 -> Delay 635/1
  Delay 876/1 -> Delay 636/1
  Delay 874/1 -> Delay 634/1
  Delay 877/1 -> Delay 637/1
  Delay 878/1 -> Delay 638/1
  Delay 879/1 -> Delay 639/1
  Delay 950/1 -> Delay 710/1
  Delay 951/1 -> Delay 711/1
  Delay 952/1 -> Delay 712/1
  Delay 953/1 -> Delay 713/1
  Delay 954/1 -> Delay 714/1
  Delay 947/1 -> Delay 707/1
  Delay 948/1 -> Delay 708/1
  Delay 949/1 -> Delay 709/1
